simulink model "PNEUMA"  (R2023b)
settings: Solver=ode23tb  StartTime=0  StopTime=3600  FixedStep=0.001  MaxStep=time_step_new  RelTol=0.01  EnableMultiTasking=on
values from neighbouring files (symbols this model uses):
  A = 20.9    [Gas_Exchange_IC.m]    (also in getPneumonia.m = (LF1-LF2)/(1-exp(Rresolve*(t2(end)-t2(1)))))
  a1 = 0.3836    [Dissociation_Spencer_IC.m]    (also in Gas_Exchange_IC.m; Respiratory_IC.m)
  a2 = 1.819    [Dissociation_Spencer_IC.m]    (also in Gas_Exchange_IC.m; Respiratory_IC.m)
  alpha1 = 0.02598    [Dissociation_Spencer_IC.m]    (also in Gas_Exchange_IC.m; Respiratory_IC.m)
  alpha2 = 0.05591    [Dissociation_Spencer_IC.m]    (also in Gas_Exchange_IC.m; Respiratory_IC.m)
  B = 92.8    [Gas_Exchange_IC.m]    (also in getPneumonia.m = LungFunction(end)-A)
  beta1 = 0.012275    [Dissociation_Spencer_IC.m]    (also in Gas_Exchange_IC.m; Respiratory_IC.m)
  beta2 = 0.03255    [Dissociation_Spencer_IC.m]    (also in Gas_Exchange_IC.m; Respiratory_IC.m)
  C = 10570    [Gas_Exchange_IC.m]
  C1 = 9    [Dissociation_Spencer_IC.m]    (also in Gas_Exchange_IC.m; Respiratory_IC.m)
  C2 = 87.00    (= 87)    [Dissociation_Spencer_IC.m]    (also in Gas_Exchange_IC.m; Respiratory_IC.m)
  Circadian_Period = 24    [Respiratory_IC.m]    (also in State_UA_Khoo_IC.m)
  CvCO2IC = 0.5116    [Body_Khoo_IC.m]    (also in Gas_Exchange_IC.m; Respiratory_IC.m = 0.5247)
  CvO2IC = 0.1672    [Body_Khoo_IC.m]    (also in Gas_Exchange_IC.m; Respiratory_IC.m = 0.1639)
  D = -5.251    [Gas_Exchange_IC.m]
  Dead1CO2IC = 0.1020    (= 0.102)    [Dead_Space_Khoo_IC.m]    (also in Gas_Exchange_IC.m; Respiratory_IC.m = 39.5616)
  Dead1O2IC = 149.8824    [Dead_Space_Khoo_IC.m]    (also in Gas_Exchange_IC.m; Respiratory_IC.m = 104.3637)
  Dead2CO2IC = 0.5274    [Dead_Space_Khoo_IC.m]    (also in Gas_Exchange_IC.m; Respiratory_IC.m = 39.6736)
  Dead2O2IC = 149.3923    [Dead_Space_Khoo_IC.m]    (also in Gas_Exchange_IC.m; Respiratory_IC.m = 104.2258)
  Dead3CO2IC = 2.2996    [Dead_Space_Khoo_IC.m]    (also in Gas_Exchange_IC.m; Respiratory_IC.m = 39.8127)
  Dead3O2IC = 147.3503    [Dead_Space_Khoo_IC.m]    (also in Gas_Exchange_IC.m; Respiratory_IC.m = 104.0505)
  Dead4CO2IC = 8.2293    [Dead_Space_Khoo_IC.m]    (also in Gas_Exchange_IC.m; Respiratory_IC.m = 40.0061)
  Dead4O2IC = 140.5179    [Dead_Space_Khoo_IC.m]    (also in Gas_Exchange_IC.m; Respiratory_IC.m = 103.8005)
  Dead5CO2IC = 22.0757    [Dead_Space_Khoo_IC.m]    (also in Gas_Exchange_IC.m; Respiratory_IC.m = 40.3359)
  Dead5O2IC = 124.5641    [Dead_Space_Khoo_IC.m]    (also in Gas_Exchange_IC.m; Respiratory_IC.m = 103.3579)
  DtotalIC = 0.3    [NeuroMuscular_IC.m]    (also in Respiratory_IC.m = 0.32)
  E_CW = 5    [Pleural_Schuessler_IC.m]    (also in Pmus_Flow_Younes_IC.m; Resp_Mech_IC.m; Respiratory_IC.m)
  E_L = 5    [Pleural_Schuessler_IC.m]    (also in Pmus_Flow_Younes_IC.m; Resp_Mech_IC.m; Respiratory_IC.m)
  fc = 0.4/60    (= 0.00666666666667)    [Respiratory_IC.m]    (also in State_UA_Khoo_IC.m)
  fcs_max = 47.78    [Cardiovascular_IC.m]    (also in Reflex_Ursino_IC.m)
  fcs_min = 2.52    [Cardiovascular_IC.m]    (also in Reflex_Ursino_IC.m)
  fcs_zero = 25    [Respiratory_IC.m]
  FlowIC = 0    [Pmus_Flow_Younes_IC.m]    (also in Resp_Mech_IC.m; Respiratory_IC.m)
  fp_inf = 6.3    [Respiratory_IC.m]
  fp_zero = 3.2    [Respiratory_IC.m]
  fs_inf = 2.10    (= 2.1)    [Respiratory_IC.m]
  fs_zero = 16.11    [Respiratory_IC.m]
  ftbs_min = 0.1    [Cardiovascular_IC.m]    (also in SA_Node_Ursino_IC.m)
  gc = 0.008/60    (= 0.000133333333333)    [Respiratory_IC.m]    (also in State_UA_Khoo_IC.m)
  h = 0.0183    [Brain_Khoo_IC.m]    (also in Gas_Exchange_IC.m; Respiratory_IC.m)
  HP_basal = 0.58    [Cardiovascular_IC.m]    (also in SA_Node_Ursino_IC.m)
  Ic = 45    [Gas_Exchange_IC.m]    (also in Respiratory_IC.m; Vent_Drive_Khoo_IC.m)
  IpCO2 = 38    [Gas_Exchange_IC.m]    (also in Respiratory_IC.m; Vent_Drive_Khoo_IC.m)
  IpO2 = 102.4    [Gas_Exchange_IC.m]    (also in Respiratory_IC.m; Vent_Drive_Khoo_IC.m)
  K1 = 13    [Dissociation_Spencer_IC.m]    (also in Gas_Exchange_IC.m; Respiratory_IC.m)
  K2 = 194.4    [Dissociation_Spencer_IC.m]    (also in Gas_Exchange_IC.m; Respiratory_IC.m)
  k_cs = 11.758    [Cardiovascular_IC.m]    (also in Reflex_Ursino_IC.m)
  k_p = 7.06    [Respiratory_IC.m]
  k_s = 0.07    [Respiratory_IC.m]
  lambda = 863    [Gas_Exchange_IC.m]    (also in Lungs_Khoo_IC.m; Respiratory_IC.m)
  Mech_Vent_pressure = 17    [Mech_vent_test.m]
  MRbCO2 = 0.0517    [Brain_Khoo_IC.m]    (also in Gas_Exchange_IC.m; Respiratory_IC.m)
  MRCO2 = 0.0033    [Body_Khoo_IC.m]    (also in Gas_Exchange_IC.m; Respiratory_IC.m)
  MRO2 = 0.0038    [Body_Khoo_IC.m]    (also in Gas_Exchange_IC.m; Respiratory_IC.m)
  NM_block_gain = 1    [Mech_vent_test.m]
  PACO2_delayIC = 39.6041    [Cardio_Mix_Lange_IC.m]    (also in Gas_Exchange_IC.m; Respiratory_IC.m = 40.4448)
  PaCO2firstIC = 0.2150    (= 0.215)    [Cardio_Mix_Lange_IC.m]    (also in Gas_Exchange_IC.m; Respiratory_IC.m = -0.2465)
  PACO2IC = 37.1484    [Gas_Exchange_IC.m]    (also in Lungs_Khoo_IC.m; Respiratory_IC.m = 40.9432)
  PaCO2secondIC = 38.4577    [Cardio_Mix_Lange_IC.m]    (also in Gas_Exchange_IC.m; Respiratory_IC.m = 40.3928)
  PAO2_delayIC = 103.8436    [Cardio_Mix_Lange_IC.m]    (also in Gas_Exchange_IC.m; Respiratory_IC.m = 103.1223)
  PaO2firstIC = -0.2838    [Cardio_Mix_Lange_IC.m]    (also in Gas_Exchange_IC.m; Respiratory_IC.m = 0.3557)
  PAO2IC = 107.1983    [Gas_Exchange_IC.m]    (also in Lungs_Khoo_IC.m; Respiratory_IC.m = 102.5153)
  PaO2secondIC = 105.4828    [Cardio_Mix_Lange_IC.m]    (also in Gas_Exchange_IC.m; Respiratory_IC.m = 103.1435)
  PbCO2IC = 48.2858    [Brain_Khoo_IC.m]    (also in Gas_Exchange_IC.m; Respiratory_IC.m = 48.5383)
  PICO2 = 0    [Dead_Space_Khoo_IC.m]    (also in Gas_Exchange_IC.m; Respiratory_IC.m)
  PIO2 = 150    [Dead_Space_Khoo_IC.m]    (also in Gas_Exchange_IC.m; Respiratory_IC.m)
  PIO2_change = -90    [Mech_vent_test.m]    (also in Respiratory_IC.m = 0)
  Pn = 90    [Cardiovascular_IC.m]    (also in Reflex_Ursino_IC.m)
  Pt_frcIC1 = 0    [Pmus_Flow_Younes_IC.m]    (also in Resp_Mech_IC.m; Respiratory_IC.m)
  Pt_frcIC2 = 0    [Pmus_Flow_Younes_IC.m]    (also in Resp_Mech_IC.m; Respiratory_IC.m)
  QdBo = 0.8333    [Brain_Khoo_IC.m]    (also in Gas_Exchange_IC.m; Respiratory_IC.m)
  R_AW = 1.27    [Pleural_Schuessler_IC.m]    (also in Pmus_Flow_Younes_IC.m; Resp_Mech_IC.m; Respiratory_IC.m)
  R_CW = 1.03    [Pleural_Schuessler_IC.m]    (also in Pmus_Flow_Younes_IC.m; Resp_Mech_IC.m; Respiratory_IC.m)
  R_L = 1.69    [Pleural_Schuessler_IC.m]    (also in Pmus_Flow_Younes_IC.m; Resp_Mech_IC.m; Respiratory_IC.m)
  RC = 0.06    [Pleural_Schuessler_IC.m]    (also in Pmus_Flow_Younes_IC.m; Resp_Mech_IC.m; Respiratory_IC.m)
  rc = 0.2/60    (= 0.00333333333333)    [Respiratory_IC.m]    (also in State_UA_Khoo_IC.m)
  SbCO2 = 0.3600    (= 0.36)    [Brain_Khoo_IC.m]    (also in Gas_Exchange_IC.m; Respiratory_IC.m)
  SCO2 = 0.0043    [Brain_Khoo_IC.m]    (also in Gas_Exchange_IC.m; Respiratory_IC.m)
  SWAo = 0.007    [Respiratory_IC.m]    (also in State_UA_Khoo_IC.m)
  T1 = 1    [Cardio_Mix_Lange_IC.m]    (also in Gas_Exchange_IC.m; Respiratory_IC.m)
  T2 = 2    [Cardio_Mix_Lange_IC.m]    (also in Gas_Exchange_IC.m; Respiratory_IC.m)
  t_end_new = 4*24*60*60    (= 345600)    [Mech_vent_test.m]
  t_end_UA = 0    [Respiratory_IC.m]    (also in State_UA_Khoo_IC.m)
  t_Mech_Vent_duration = 0    [Mech_vent_test.m]
  t_Mech_Vent_start = 0    [Mech_vent_test.m]
  t_Mueller_duration = 0    [NeuroMuscular_IC.m]
  t_Mueller_insp = 0    [NeuroMuscular_IC.m]
  t_Mueller_start = 0    [NeuroMuscular_IC.m]
  t_NM_block_duration = 0    [Mech_vent_test.m]
  t_NM_block_start = 0    [Mech_vent_test.m]
  t_O2_duration = 0    [Mech_vent_test.m]    (also in Respiratory_IC.m)
  t_O2_start = 0    [Mech_vent_test.m]    (also in Respiratory_IC.m)
  t_start_new = 0    [Mech_vent_test.m]
  t_start_UA = 0    [Respiratory_IC.m]    (also in State_UA_Khoo_IC.m)
  t_valsalva_duration = 0    [NeuroMuscular_IC.m]
  t_valsalva_insp = 0    [NeuroMuscular_IC.m]
  t_valsalva_start = 0    [NeuroMuscular_IC.m]
  time_step = time_step    [acquire_data.m]    (also in acquire_data_save.m)
  VC = 5    [Pmus_Flow_Younes_IC.m]    (also in Resp_Mech_IC.m; Respiratory_IC.m)
  Vdead1 = 0.03    [Dead_Space_Khoo_IC.m]    (also in Gas_Exchange_IC.m; Respiratory_IC.m)
  Vdead2 = 0.03    [Dead_Space_Khoo_IC.m]    (also in Gas_Exchange_IC.m; Respiratory_IC.m)
  Vdead3 = 0.03    [Dead_Space_Khoo_IC.m]    (also in Gas_Exchange_IC.m; Respiratory_IC.m)
  Vdead4 = 0.03    [Dead_Space_Khoo_IC.m]    (also in Gas_Exchange_IC.m; Respiratory_IC.m)
  Vdead5 = 0.03    [Dead_Space_Khoo_IC.m]    (also in Gas_Exchange_IC.m; Respiratory_IC.m)
  Ventilator_rate = 12    [Mech_vent_test.m]
  VTCO2 = 15    [Body_Khoo_IC.m]    (also in Gas_Exchange_IC.m; Respiratory_IC.m)
  VtIC = 0    [Pmus_Flow_Younes_IC.m]    (also in Resp_Mech_IC.m; Respiratory_IC.m)
  VTO2 = 6    [Body_Khoo_IC.m]    (also in Gas_Exchange_IC.m; Respiratory_IC.m)
  Z = 0.0227    [Dissociation_Spencer_IC.m]    (also in Gas_Exchange_IC.m; Respiratory_IC.m)
undefined symbols (not defined in the file or in its folder): A_0_ua, alpha_E_FFA_Heart, alpha_E_FFA_muscle, alpha_E_GLC_Heart, alpha_E_GLC_muscle, alpha_E_GLY_muscle, alpha_E_PYR_muscle, alpha_E_TGL_adipose, alpha_E_TGL_GI, alpha_E_TGL_Heart, alpha_E_TGL_muscle, Arousal_UAIC, C_ua_awake, Cbp, Cbv, Ce_0, Cep, Cev, Chp, Chv, Cla, Clamp_class, Cmp, Cmv, Cpa, CPAP_pressure, Cpp, Cpv, Cra, Csa, Csp, Csv, CvbO2_n, CvhO2_n, CvmO2_n, DAY, delay, DietBlock, Dx, Fb, fchemo_max, fchemo_min, fchemoIC, flsIC, Ftas_I0, ftas_min, ftas_r0, FVC_activation, gain_E, Gamma, Gas_sleep, Gas_sleepM, Gb, Gblock, GbO2, Gbs_sleep, gcc_sa, gcc_sb, gcc_sp, Gclamp ... (+144)
libraries: simulink x4, dspstat3 x4, simulink_extras x2
(part 7 of 8)

== system PNEUMA/Metabolic Control/Epinephrine Regulation on Heart and Muscle/Epi Modulation/Muscle ==
  Ce(t) : Inport
  Add : Sum  Inputs=+++++
  Fcn{,1..4} (5 alike) : Fcn  Expr=u(2) * ( 1+ u(4) * (u(1) - u(3))^2/( u(5)+(u(1) - u(3))^2 ))
  Muscle: FFA_to_ACoA : Constant  Value=[V_0_FFA_muscle, Ce_0, lamda_E_FFA_muscle, alpha_E_FFA_muscle]
  Muscle: GLC_to_G6P : Constant  Value=[V_0_GLC_muscle, Ce_0, lamda_E_GLC_muscle, alpha_E_GLC_muscle]
  Muscle: GLY_to_G6P : Constant  Value=[V_0_GLY_muscle, Ce_0, lamda_E_GLY_muscle, alpha_E_GLY_muscle]
  Muscle: PYR_to_ALA : Constant  Value=[V_0_PYR_muscle, Ce_0, lamda_E_PYR_muscle, alpha_E_PYR_muscle]
  Muscle: TGL_to_FFA : Constant  Value=[V_0_TGL_muscle, Ce_0, lamda_E_TGL_muscle, alpha_E_TGL_muscle]
  Mux{,1..2,4..5} (5 alike) : Mux  Inputs=2
  Mux3 : Mux  Inputs=5
  Epi on Muscle (Fluxes) : Outport
  Epi on Muscle(Sum) : Outport  Port=2
  wires:
  Ce(t)/1 -> Mux/1, Mux1/1, Mux2/1, Mux4/1, Mux5/1
  Muscle: GLC_to_G6P/1 -> Mux/2
  Mux/1 -> Fcn/1
  Muscle: GLY_to_G6P/1 -> Mux1/2
  Mux1/1 -> Fcn1/1
  Muscle: FFA_to_ACoA/1 -> Mux2/2
  Mux2/1 -> Fcn2/1
  Fcn/1 -> Mux3/1, Add/1
  Fcn1/1 -> Mux3/2, Add/2
  Muscle: TGL_to_FFA/1 -> Mux4/2
  Mux4/1 -> Fcn3/1
  Fcn3/1 -> Mux3/5, Add/5
  Fcn2/1 -> Mux3/3, Add/3
  Mux3/1 -> Epi on Muscle (Fluxes)/1
  Add/1 -> Epi on Muscle(Sum)/1
  Muscle: PYR_to_ALA/1 -> Mux5/2
  Mux5/1 -> Fcn4/1
  Fcn4/1 -> Mux3/4, Add/4

== system PNEUMA/Metabolic Control/Glucose-Insulin-FFA Minimal Model/Saving deltaFtas_WalphaSYMP/Switch Case Action Subsystem ==
  In1 : Inport
  Action Port : ActionPort  ActionPortLabel=case [ 0 ]:
  To File : ToFile  Filename=deltaFtas1.mat  MatrixName=deltaFtas  SampleTime=sampletime
  wires:
  In1/1 -> To File/1

== system PNEUMA/Metabolic Control/Glucose-Insulin-FFA Minimal Model/Saving deltaFtas_WalphaSYMP/Switch Case Action Subsystem1 ==
  In1 : Inport
  Action Port : ActionPort  ActionPortLabel=case [ 1 ]:
  To File : ToFile  Filename=deltaFtas2.mat  MatrixName=deltaFtas  SampleTime=sampletime
  wires:
  In1/1 -> To File/1

== system PNEUMA/Metabolic Control/Glucose-Insulin-FFA Minimal Model/Saving deltaFtas_WalphaSYMP/Switch Case Action Subsystem2 ==
  In1 : Inport
  Action Port : ActionPort  ActionPortLabel=case [ 2 ]:
  To File : ToFile  Filename=deltaFtas3.mat  MatrixName=deltaFtas  SampleTime=sampletime
  wires:
  In1/1 -> To File/1

== system PNEUMA/Metabolic Control/Glucose-Insulin-FFA Minimal Model/Saving deltaFtas_WalphaSYMP/Switch Case Action Subsystem3 ==
  In1 : Inport
  Action Port : ActionPort  ActionPortLabel=default:
  To File : ToFile  Filename=deltaFtas10.mat  MatrixName=deltaFtas  SampleTime=sampletime
  wires:
  In1/1 -> To File/1

== system PNEUMA/Metabolic Control/Glucose-Insulin-FFA Minimal Model/Saving deltaFtas_WalphaSYMP/Switch Case Action Subsystem4 ==
  In1 : Inport
  Action Port : ActionPort  ActionPortLabel=case [ 3 ]:
  To File : ToFile  Filename=deltaFtas4.mat  MatrixName=deltaFtas  SampleTime=sampletime
  wires:
  In1/1 -> To File/1

== system PNEUMA/Metabolic Control/Glucose-Insulin-FFA Minimal Model/Saving deltaFtas_WalphaSYMP/Switch Case Action Subsystem5 ==
  In1 : Inport
  Action Port : ActionPort  ActionPortLabel=case [ 4 ]:
  To File : ToFile  Filename=deltaFtas5.mat  MatrixName=deltaFtas  SampleTime=sampletime
  wires:
  In1/1 -> To File/1

== system PNEUMA/Metabolic Control/Glucose-Insulin-FFA Minimal Model/Saving deltaFtas_WalphaSYMP/Switch Case Action Subsystem6 ==
  In1 : Inport
  Action Port : ActionPort  ActionPortLabel=case [ 5 ]:
  To File : ToFile  Filename=deltaFtas6.mat  MatrixName=deltaFtas  SampleTime=sampletime
  wires:
  In1/1 -> To File/1

== system PNEUMA/Metabolic Control/Glucose-Insulin-FFA Minimal Model/Saving deltaFtas_WalphaSYMP/Switch Case Action Subsystem7 ==
  In1 : Inport
  Action Port : ActionPort  ActionPortLabel=case [ 6 ]:
  To File : ToFile  Filename=deltaFtas7.mat  MatrixName=deltaFtas  SampleTime=sampletime
  wires:
  In1/1 -> To File/1

== system PNEUMA/Metabolic Control/Glucose-Insulin-FFA Minimal Model/Saving deltaFtas_WalphaSYMP/Switch Case Action Subsystem8 ==
  In1 : Inport
  Action Port : ActionPort  ActionPortLabel=case [ 7 ]:
  To File : ToFile  Filename=deltaFtas8.mat  MatrixName=deltaFtas  SampleTime=sampletime
  wires:
  In1/1 -> To File/1

== system PNEUMA/Metabolic Control/Glucose-Insulin-FFA Minimal Model/Saving deltaFtas_WalphaSYMP/Switch Case Action Subsystem9 ==
  In1 : Inport
  Action Port : ActionPort  ActionPortLabel=case [ 8 ]:
  To File : ToFile  Filename=deltaFtas9.mat  MatrixName=deltaFtas  SampleTime=sampletime
  wires:
  In1/1 -> To File/1

== system PNEUMA/Respiratory System/Gas Exchange/BODY TISSUES COMPARTMENT/Body Tissues Compartment for CO2 ==
  CaCO2 : Inport
  Qt : Inport  Port=2
  SI Sleep Wake State Index : Inport  Port=3
  Fcn : Fcn  Expr=MRCO2*(0.375*(1-0.4*u)+0.625)
  Fcn -5 blocks : Fcn  Expr=( u(1) + ( u(2) * u(3)) ) /VTCO2
  Integrator : Integrator  InitialCondition=CvCO2IC
  Mux : Mux  Inputs=3
  Sum1 : Sum  Inputs=+-  InputSameDT=on  SaturateOnIntegerOverflow=on  OutDataTypeStr=Inherit: Same as first input
  CvCO2 : Outport
  tag scope: CvCO2IC=global
  wires:
  SI Sleep Wake State Index/1 -> Fcn/1
  CaCO2/1 -> Sum1/1
  Fcn -5 blocks/1 -> Integrator/1
  Integrator/1 -> [CvCO2IC], Sum1/2, CvCO2/1
  Mux/1 -> Fcn -5 blocks/1
  Fcn/1 -> Mux/1
  Qt/1 -> Mux/2
  Sum1/1 -> Mux/3

== system PNEUMA/Respiratory System/Gas Exchange/BODY TISSUES COMPARTMENT/Body Tissues Compartment for O2 ==
  Qt : Inport
  SI Sleep Wake State Index : Inport  Port=2
  CaO2 : Inport  Port=3
  Fcn : Fcn  Expr=MRO2*(0.375*(1-0.4*u)+0.625)
  Fcn -5 blocks : Fcn  Expr=( -u(1) + ( u(2) * u(3)) ) /VTO2
  Integrator : Integrator  InitialCondition=CvO2IC
  Mux : Mux  Inputs=3
  Sum1 : Sum  Inputs=+-  InputSameDT=on  SaturateOnIntegerOverflow=on  OutDataTypeStr=Inherit: Same as first input
  CVO2 : Outport
  tag scope: CvO2IC=global
  wires:
  SI Sleep Wake State Index/1 -> Fcn/1
  Qt/1 -> Mux/2
  Sum1/1 -> Mux/3
  CaO2/1 -> Sum1/1
  Fcn -5 blocks/1 -> Integrator/1
  Integrator/1 -> [CvO2IC], Sum1/2, CVO2/1
  Mux/1 -> Fcn -5 blocks/1
  Fcn/1 -> Mux/1

== system PNEUMA/Respiratory System/Gas Exchange/Cardiovascular Mixing and Convection/CO2 Cardiovascular Mixing and Convection Effects ==
  PACO2 : Inport
  Q : Inport  Port=2
  Lung-Chemoreceptor Delay Volume : Inport  Port=3
  1/(T1*T2) : Gain  Gain=1/(T1*T2)  SaturateOnIntegerOverflow=on  OutDataTypeStr=Inherit: Same as input  ParamDataTypeStr=Inherit: Same as input
  Integrator : Integrator  InitialCondition=PaCO2firstIC
  Integrator1 : Integrator  InitialCondition=PaCO2secondIC
  PACO2 delay : VariableTransportDelay  MaximumDelay=100  InitialOutput=PACO2_delayIC  MaximumPoints=22528
  Product1 : Product  Inputs=*/  InputSameDT=on  SaturateOnIntegerOverflow=on  OutDataTypeStr=Inherit: Same as first input
  Sum : Sum  Inputs=--+  InputSameDT=on  SaturateOnIntegerOverflow=on  OutDataTypeStr=Inherit: Same as first input
  T1+T2 : Gain  Gain=T1+T2  SaturateOnIntegerOverflow=on  OutDataTypeStr=Inherit: Same as input  ParamDataTypeStr=Inherit: Same as input
  PaCO2 : Outport
  tag scope: PACO2_delayIC=global, PaCO2firstIC=global, PaCO2secondIC=global
  wires:
  T1+T2/1 -> Sum/1
  Integrator/1 -> T1+T2/1, Integrator1/1, [PaCO2firstIC]
  Sum/1 -> 1/(T1*T2)/1
  1/(T1*T2)/1 -> Integrator/1
  Integrator1/1 -> Sum/2, [PaCO2secondIC], PaCO2/1
  PACO2/1 -> PACO2 delay/1
  PACO2 delay/1 -> [PACO2_delayIC], Sum/3
  Product1/1 -> PACO2 delay/2
  Lung-Chemoreceptor Delay Volume/1 -> Product1/1
  Q/1 -> Product1/2

== system PNEUMA/Respiratory System/Gas Exchange/Cardiovascular Mixing and Convection/O2 Cardiovascular Mixing and Convection Effects ==
  note: Warning: Division by zero in block 'pneuma_cardiovascular/Respiratory_System/Gas Exchange/Cardiovascular Mixing and Convection/O2 Cardiovascular Mixing and Convection Effects/PAO2 Save Subsystem/Product1'.
  Q : Inport
  PAO2 : Inport  Port=2
  Lung-Chemoreceptor Delay Volume : Inport  Port=3
  1/(T1*T2) : Gain  Gain=1/(T1*T2)  SaturateOnIntegerOverflow=on  OutDataTypeStr=Inherit: Same as input  ParamDataTypeStr=Inherit: Same as input
  Integrator : Integrator  InitialCondition=PaO2firstIC
  Integrator1 : Integrator  InitialCondition=PaO2secondIC
  PAO2 delay : VariableTransportDelay  MaximumDelay=100  InitialOutput=PAO2_delayIC  MaximumPoints=22528
  Product1 : Product  Inputs=*/  InputSameDT=on  SaturateOnIntegerOverflow=on  OutDataTypeStr=Inherit: Same as first input
  Sum : Sum  Inputs=+--  InputSameDT=on  SaturateOnIntegerOverflow=on  OutDataTypeStr=Inherit: Same as first input
  T1+T2 : Gain  Gain=T1+T2  SaturateOnIntegerOverflow=on  OutDataTypeStr=Inherit: Same as input  ParamDataTypeStr=Inherit: Same as input
  PaO2 : Outport
  tag scope: PAO2_delayIC=global, PaO2firstIC=global, PaO2secondIC=global
  wires:
  1/(T1*T2)/1 -> Integrator/1
  Sum/1 -> 1/(T1*T2)/1
  Integrator/1 -> Integrator1/1, T1+T2/1, [PaO2firstIC]
  Integrator1/1 -> Sum/2, PaO2/1, [PaO2secondIC]
  T1+T2/1 -> Sum/3
  Product1/1 -> PAO2 delay/2
  PAO2/1 -> PAO2 delay/1
  PAO2 delay/1 -> [PAO2_delayIC], Sum/1
  Lung-Chemoreceptor Delay Volume/1 -> Product1/1
  Q/1 -> Product1/2

== system PNEUMA/Respiratory System/Gas Exchange/DEAD SPACE/CO2 DEAD SPACE ==
  PACO2 : Inport
  Flow : Inport  Port=2
  Constant : Constant  Value=PICO2
  Pd(1)CO2 : Subsystem
  Pd(2)CO2 : Subsystem
  Pd(3)CO2 : Subsystem
  Pd(4)CO2 : Subsystem
  Pd(5)CO2 : Subsystem
  Pd5CO2 : Outport
  tag scope: BreathCO2=global
  wires:
  Pd(4)CO2/1(Pd(4)CO2) -> Pd(3)CO2/3(Pd(4)CO2), Pd(5)CO2/1(Pd(4)CO2)
  Pd(3)CO2/1(Pd(3)CO2) -> Pd(4)CO2/1(Pd(3)CO2), Pd(2)CO2/3(Pd(3)CO2)
  Pd(2)CO2/1(Pd(2)CO2) -> Pd(3)CO2/1(Pd(2)CO2), Pd(1)CO2/3(Pd(2)CO2)
  Pd(1)CO2/1(Pd(1)CO2) -> [BreathCO2], Pd(2)CO2/1(Pd(1)CO2)
  Flow/1 -> Pd(1)CO2/2(Flow), Pd(2)CO2/2(Flow), Pd(4)CO2/2(Flow), Pd(5)CO2/2(Flow), Pd(3)CO2/2(Flow)
  PACO2/1 -> Pd(5)CO2/3(PACO2)
  Pd(5)CO2/1(Pd(5)CO2) -> Pd5CO2/1, Pd(4)CO2/3(Pd(5)CO2)
  Constant/1 -> Pd(1)CO2/1(PICO2)

== system PNEUMA/Respiratory System/Gas Exchange/DEAD SPACE/O2 DEAD SPACE ==
  Flow : Inport
  PAO2 : Inport  Port=2
  Pd(1)O2 : Subsystem
  Pd(2)O2 : Subsystem
  Pd(3)O2 : Subsystem
  Pd(4)O2 : Subsystem
  Pd(5)O2 : Subsystem
  Pd5O2 : Outport
  wires:
  Pd(4)O2/1(Pd(4)O2) -> Pd(3)O2/3(Pd(4)O2), Pd(5)O2/1(Pd(4)O2)
  Pd(3)O2/1(Pd(3)O2) -> Pd(4)O2/1(Pd(3)O2), Pd(2)O2/3(Pd(3)O2)
  Pd(2)O2/1(Pd(2)O2) -> Pd(3)O2/1(Pd(2)O2), Pd(1)O2/3(Pd(2)O2)
  Pd(1)O2/1(Pd(1)O2) -> Pd(2)O2/1(Pd(1)O2)
  PAO2/1 -> Pd(5)O2/3(PAO2)
  Flow/1 -> Pd(4)O2/2(Flow), Pd(5)O2/2(Flow), Pd(2)O2/2(Flow), Pd(1)O2/2(Flow), Pd(3)O2/2(Flow)
  Pd(5)O2/1(Pd(5)O2) -> Pd5O2/1, Pd(4)O2/3(Pd(5)O2)
  [PIO2] -> Pd(1)O2/1(PIO2)

== system PNEUMA/Respiratory System/Gas Exchange/GAS EXCHANGE IN THE LUNGS/CO2 Gas Exchange in the Lungs ==
  CaCO2 : Inport
  CVCO2 : Inport  Port=2
  Pd5CO2 : Inport  Port=3
  Vt - Tidal Volume : Inport  Port=4
  Flow : Inport  Port=5
  "Q " : Inport  Port=6
  Constant : Constant  Value=lambda
  Fcn -11 blocks : Fcn  Expr=(((u(2) >=0) * u(2) * u(1) + (u(2) <0) * 0 ) + (u(3) - u(4)) *u(5) * ( u(7)*(1-s) ) )/( u(6)+VLCO2)
  From Workspace : FromWorkspace  VariableName=LungFunction
  Integrator : Integrator  InitialCondition=PACO2IC
  Mux : Mux  Inputs=7
  Product : Product  Inputs=*/
  sum1 : Sum  Inputs=-+  InputSameDT=on  SaturateOnIntegerOverflow=on  OutDataTypeStr=Inherit: Same as first input
  PACO2 : Outport
  tag scope: PACO2IC=global
  wires:
  "Q "/1 -> Mux/5
  CVCO2/1 -> Mux/3
  CaCO2/1 -> Mux/4
  Fcn -11 blocks/1 -> Integrator/1
  Integrator/1 -> [PACO2IC], PACO2/1, sum1/1
  Pd5CO2/1 -> sum1/2
  Mux/1 -> Fcn -11 blocks/1
  sum1/1 -> Mux/1
  Flow/1 -> Mux/2
  Vt - Tidal Volume/1 -> Mux/6
  Product/1 -> Mux/7
  Constant/1 -> Product/1
  From Workspace/1 -> Product/2

== system PNEUMA/Respiratory System/Gas Exchange/GAS EXCHANGE IN THE LUNGS/O2 Gas Exchange in the Lungs ==
  Vt - Tidal Volume : Inport
  Flow : Inport  Port=2
  Q : Inport  Port=3
  CaO2 : Inport  Port=4
  CVO2 : Inport  Port=5
  Pd5O2 : Inport  Port=6
  Constant : Constant  Value=lambda
  Fcn -11 blocks : Fcn  Expr=(((u(2) >=0) * u(2) * u(1) + (u(2) <0) * 0 ) + (u(4) - u(5)) *u(3) * ( u(7)*(1-s) ) )/( u(6)+VLO2 )
  From Workspace : FromWorkspace  VariableName=LungFunction
  Integrator : Integrator  InitialCondition=PAO2IC  LimitOutput=on  LowerSaturationLimit=0
  Mux : Mux  Inputs=7
  Product : Product  Inputs=*/
  Sum2 : Sum  Inputs=-+  InputSameDT=on  SaturateOnIntegerOverflow=on  OutDataTypeStr=Inherit: Same as first input
  PAO2 : Outport
  tag scope: LungFunction=global, PAO2IC=global
  wires:
  Integrator/1 -> PAO2/1, [PAO2IC], Sum2/1
  Fcn -11 blocks/1 -> Integrator/1
  Pd5O2/1 -> Sum2/2
  Mux/1 -> Fcn -11 blocks/1
  Sum2/1 -> Mux/1
  Flow/1 -> Mux/2
  Q/1 -> Mux/3
  CVO2/1 -> Mux/4
  CaO2/1 -> Mux/5
  Vt - Tidal Volume/1 -> Mux/6
  Product/1 -> Mux/7
  Constant/1 -> Product/1
  From Workspace/1 -> [LungFunction], Product/2

== system PNEUMA/Respiratory System/Respiratory_Mechanics/Pleural_Pressure1/Pa ==
  "Flow " : Inport
  "Pao " : Inport  Port=2
  Fcn : Fcn  Expr=(u>=0)*u * (kaw1 + abs( (u>=0)*u) *kaw2)
  Fcn1 : Fcn  Expr=(u>=0)*u
  Sum2 : Sum  Inputs=+-  InputSameDT=on  SaturateOnIntegerOverflow=on  OutDataTypeStr=Inherit: Same as first input
  "Pa " : Outport
  wires:
  "Flow "/1 -> Fcn/1
  "Pao "/1 -> Sum2/1
  Sum2/1 -> Fcn1/1
  Fcn/1 -> Sum2/2
  Fcn1/1 -> "Pa "/1

== system PNEUMA/Respiratory System/Respiratory_Mechanics/Pleural_Pressure1/Pcw ==
  Vt : Inport
  Flow : Inport  Port=2
  Fcn : Fcn  Expr=(u>=0)*u
  Pcw_0 : Constant  Value=-1
  Product3 : Product  InputSameDT=on  SaturateOnIntegerOverflow=on  OutDataTypeStr=Inherit: Same as first input
  Product4 : Product  InputSameDT=on  SaturateOnIntegerOverflow=on  OutDataTypeStr=Inherit: Same as first input
  Sum3 : Sum  Inputs=+++  InputSameDT=on  SaturateOnIntegerOverflow=on  OutDataTypeStr=Inherit: Same as first input
  elastance : Constant  Value=E_CW
  "resistance " : Constant  Value=R_CW
  "Pcw " : Outport
  wires:
  Fcn/1 -> Product3/2
  Vt/1 -> Product4/1
  elastance/1 -> Product4/2
  Sum3/1 -> "Pcw "/1
  Product4/1 -> Sum3/2
  Flow/1 -> Fcn/1
  Product3/1 -> Sum3/1
  "resistance "/1 -> Product3/1
  Pcw_0/1 -> Sum3/3

== system PNEUMA/Respiratory System/Respiratory_Mechanics/Respiratory Muscles Activity1/Resp Muscle Reaction ==
  RespMus Drive : Inport
  Step Size : Inport  Port=2
  0.735539 : Gain
  Fcn : Fcn  Expr=u(1) + u(2) + (u(2) *u(5)/u(4) - u(3)+u(1)) * (exp(-u(4)/u(5)) - 1)
  Memory : Memory  InitialCondition=Pt_frcIC1  InheritSampleTime=on
  Memory1 : Memory  InitialCondition=Pt_frcIC2  InheritSampleTime=on  LinearizeMemory=on
  Mux : Mux  Inputs=5
  RC1 : Constant  Value=RC
  Sum4 : Sum  Inputs=+-  InputSameDT=on  SaturateOnIntegerOverflow=on  OutDataTypeStr=Inherit: Same as first input
  Pt_frc : Outport
  wires:
  RespMus Drive/1 -> Sum4/1, Memory/1
  Sum4/1 -> Mux/2
  RC1/1 -> Mux/5
  Step Size/1 -> Mux/4
  Memory1/1 -> Mux/1
  Memory/1 -> Sum4/2, Mux/3
  Mux/1 -> Fcn/1
  Fcn/1 -> 0.735539/1
  0.735539/1 -> Pt_frc/1, Memory1/1

== system PNEUMA/Respiratory System/Respiratory_Mechanics/Respiratory Muscles Activity1/flow generation ==
  "Cond " : Inport
  "Pao " : Inport  Port=2
  PE : Inport  Port=3
  "Po_vt " : Inport  Port=4
  b_vt : Inport  Port=5
  Vt : Inport  Port=6
  0.25 : Gain  Gain=0.25  SaturateOnIntegerOverflow=on  OutDataTypeStr=Inherit: Same as input  ParamDataTypeStr=Inherit: Same as input
  4 : Gain  Gain=4  SaturateOnIntegerOverflow=on  OutDataTypeStr=Inherit: Same as input  ParamDataTypeStr=Inherit: Same as input
  Gain3 : Gain  Gain=1/2  SaturateOnIntegerOverflow=on  OutDataTypeStr=Inherit: Same as input  ParamDataTypeStr=Inherit: Same as input
  Math Function : Math  Operator=square  SignedPower=on
  Math Function1 : Math  Operator=sqrt  SignedPower=on
  Memory3 : Memory  InitialCondition=FlowIC  InheritSampleTime=on
  Product : Product  InputSameDT=on  SaturateOnIntegerOverflow=on  OutDataTypeStr=Inherit: Same as first input
  Product1 : Product  InputSameDT=on  SaturateOnIntegerOverflow=on  OutDataTypeStr=Inherit: Same as first input
  Product2 : Product  Inputs=3  InputSameDT=on  SaturateOnIntegerOverflow=on  OutDataTypeStr=Inherit: Same as first input
  Sum4 : Sum  Inputs=+++-  InputSameDT=on  SaturateOnIntegerOverflow=on  OutDataTypeStr=Inherit: Same as first input
  Sum5 : Sum  InputSameDT=on  SaturateOnIntegerOverflow=on  OutDataTypeStr=Inherit: Same as first input
  Sum6 : Sum  Inputs=+-  InputSameDT=on  SaturateOnIntegerOverflow=on  OutDataTypeStr=Inherit: Same as first input
  Sum7 : Sum  Inputs=++--  InputSameDT=on  SaturateOnIntegerOverflow=on  OutDataTypeStr=Inherit: Same as first input
  Sum8 : Sum  Inputs=-+  InputSameDT=on  SaturateOnIntegerOverflow=on  OutDataTypeStr=Inherit: Same as first input
  elastance : Gain  Gain=(E_CW+E_L)  SaturateOnIntegerOverflow=on  OutDataTypeStr=Inherit: Same as input  ParamDataTypeStr=Inherit: Same as input
  total_resp conductance : Constant  Value=1/(R_AW+R_L+R_CW)*1.8
  Flow : Outport
  wires:
  0.25/1 -> Sum4/1
  total_resp conductance/1 -> Product1/2
  "Cond "/1 -> Product1/1
  Product1/1 -> 4/1, Product/1
  Gain3/1 -> Memory3/1
  Sum8/1 -> Gain3/1
  Sum5/1 -> Sum8/1, Math Function/1
  Math Function1/1 -> Sum8/2
  Sum6/1 -> Math Function1/1
  Product2/1 -> Sum6/2
  "Po_vt "/1 -> Sum7/4, 0.25/1
  "Pao "/1 -> Sum7/3, Sum4/4
  PE/1 -> Sum7/2, Sum4/3
  elastance/1 -> Sum7/1, Sum4/2
  Sum7/1 -> Product2/3
  b_vt/1 -> Product2/2, Sum5/2
  4/1 -> Product2/1
  Math Function/1 -> Sum6/1
  Product/1 -> Sum5/1
  Sum4/1 -> Product/2
  Vt/1 -> elastance/1
  Memory3/1 -> Flow/1

== system PNEUMA/Respiratory System/Respiratory_Mechanics/Respiratory Muscles Activity1/flow generation 1 ==
  Po_vt_1 : Inport
  Vt_1 : Inport  Port=2
  b_vt_1 : Inport  Port=3
  PE_1 : Inport  Port=4
  Pao_1 : Inport  Port=5
  "Cond " : Inport  Port=6
  0.25 : Gain  Gain=0.25  SaturateOnIntegerOverflow=on  OutDataTypeStr=Inherit: Same as input  ParamDataTypeStr=Inherit: Same as input
  4 : Gain  Gain=4  SaturateOnIntegerOverflow=on  OutDataTypeStr=Inherit: Same as input  ParamDataTypeStr=Inherit: Same as input
  Gain3 : Gain  Gain=0.5  SaturateOnIntegerOverflow=on  OutDataTypeStr=Inherit: Same as input  ParamDataTypeStr=Inherit: Same as input
  Math Function : Math  Operator=square  SignedPower=on
  Math Function1 : Math  Operator=sqrt  SignedPower=on
  Memory1 : Memory  InitialCondition=FlowIC  InheritSampleTime=on
  Product : Product  InputSameDT=on  SaturateOnIntegerOverflow=on  OutDataTypeStr=Inherit: Same as first input
  Product1 : Product  InputSameDT=on  SaturateOnIntegerOverflow=on  OutDataTypeStr=Inherit: Same as first input
  Product2 : Product  Inputs=3  InputSameDT=on  SaturateOnIntegerOverflow=on  OutDataTypeStr=Inherit: Same as first input
  Sum4 : Sum  Inputs=+++-  InputSameDT=on  SaturateOnIntegerOverflow=on  OutDataTypeStr=Inherit: Same as first input
  Sum5 : Sum  InputSameDT=on  SaturateOnIntegerOverflow=on  OutDataTypeStr=Inherit: Same as first input
  Sum6 : Sum  Inputs=+-  InputSameDT=on  SaturateOnIntegerOverflow=on  OutDataTypeStr=Inherit: Same as first input
  Sum7 : Sum  Inputs=++--  InputSameDT=on  SaturateOnIntegerOverflow=on  OutDataTypeStr=Inherit: Same as first input
  Sum8 : Sum  Inputs=-+  InputSameDT=on  SaturateOnIntegerOverflow=on  OutDataTypeStr=Inherit: Same as first input
  elastance : Gain  Gain=(E_CW+E_L)  SaturateOnIntegerOverflow=on  OutDataTypeStr=Inherit: Same as input  ParamDataTypeStr=Inherit: Same as input
  total_resp conductance : Constant  Value=1/(R_AW+R_L+R_CW)*1.8
  Flow_1 : Outport
  wires:
  Vt_1/1 -> elastance/1
  Sum4/1 -> Product/2
  Product/1 -> Sum5/1
  Math Function/1 -> Sum6/1
  4/1 -> Product2/1
  b_vt_1/1 -> Sum5/2, Product2/2
  Sum7/1 -> Product2/3
  elastance/1 -> Sum4/2, Sum7/1
  PE_1/1 -> Sum4/3, Sum7/2
  Pao_1/1 -> Sum4/4, Sum7/3
  Po_vt_1/1 -> 0.25/1, Sum7/4
  Product2/1 -> Sum6/2
  Sum6/1 -> Math Function1/1
  Math Function1/1 -> Sum8/2
  Sum5/1 -> Math Function/1, Sum8/1
  Sum8/1 -> Gain3/1
  Gain3/1 -> Memory1/1
  Product1/1 -> Product/1, 4/1
  "Cond "/1 -> Product1/1
  total_resp conductance/1 -> Product1/2
  0.25/1 -> Sum4/1
  Memory1/1 -> Flow_1/1

== system PNEUMA/Respiratory System/Sleep Mechanism/Saving CircadianProcess/Switch Case Action Subsystem ==
  In1 : Inport
  Action Port : ActionPort  ActionPortLabel=case [ 0 ]:
  To File : ToFile  Filename=CircadianProcess1.mat  MatrixName=H_L_CircardianLow_RBM_SWA  SampleTime=sampletime
  wires:
  In1/1 -> To File/1

== system PNEUMA/Respiratory System/Sleep Mechanism/Saving CircadianProcess/Switch Case Action Subsystem1 ==
  In1 : Inport
  Action Port : ActionPort  ActionPortLabel=case [ 1 ]:
  To File : ToFile  Filename=CircadianProcess2.mat  MatrixName=H_L_CircardianLow_RBM_SWA  SampleTime=sampletime
  wires:
  In1/1 -> To File/1

== system PNEUMA/Respiratory System/Sleep Mechanism/Saving CircadianProcess/Switch Case Action Subsystem2 ==
  In1 : Inport
  Action Port : ActionPort  ActionPortLabel=case [ 2 ]:
  To File : ToFile  Filename=CircadianProcess3.mat  MatrixName=H_L_CircardianLow_RBM_SWA  SampleTime=sampletime
  wires:
  In1/1 -> To File/1

== system PNEUMA/Respiratory System/Sleep Mechanism/Saving CircadianProcess/Switch Case Action Subsystem3 ==
  In1 : Inport
  Action Port : ActionPort  ActionPortLabel=default:
  To File : ToFile  Filename=CircadianProcess10.mat  MatrixName=H_L_CircardianLow_RBM_SWA  SampleTime=sampletime
  wires:
  In1/1 -> To File/1

== system PNEUMA/Respiratory System/Sleep Mechanism/Saving CircadianProcess/Switch Case Action Subsystem4 ==
  In1 : Inport
  Action Port : ActionPort  ActionPortLabel=case [ 3 ]:
  To File : ToFile  Filename=CircadianProcess4.mat  MatrixName=H_L_CircardianLow_RBM_SWA  SampleTime=sampletime
  wires:
  In1/1 -> To File/1

== system PNEUMA/Respiratory System/Sleep Mechanism/Saving CircadianProcess/Switch Case Action Subsystem5 ==
  In1 : Inport
  Action Port : ActionPort  ActionPortLabel=case [ 4 ]:
  To File : ToFile  Filename=CircadianProcess5.mat  MatrixName=H_L_CircardianLow_RBM_SWA  SampleTime=sampletime
  wires:
  In1/1 -> To File/1

== system PNEUMA/Respiratory System/Sleep Mechanism/Saving CircadianProcess/Switch Case Action Subsystem6 ==
  In1 : Inport
  Action Port : ActionPort  ActionPortLabel=case [ 5 ]:
  To File : ToFile  Filename=CircadianProcess6.mat  MatrixName=H_L_CircardianLow_RBM_SWA  SampleTime=sampletime
  wires:
  In1/1 -> To File/1

== system PNEUMA/Respiratory System/Sleep Mechanism/Saving CircadianProcess/Switch Case Action Subsystem7 ==
  In1 : Inport
  Action Port : ActionPort  ActionPortLabel=case [ 6 ]:
  To File : ToFile  Filename=CircadianProcess7.mat  MatrixName=H_L_CircardianLow_RBM_SWA  SampleTime=sampletime
  wires:
  In1/1 -> To File/1

== system PNEUMA/Respiratory System/Sleep Mechanism/Saving CircadianProcess/Switch Case Action Subsystem8 ==
  In1 : Inport
  Action Port : ActionPort  ActionPortLabel=case [ 7 ]:
  To File : ToFile  Filename=CircadianProcess8.mat  MatrixName=H_L_CircardianLow_RBM_SWA  SampleTime=sampletime
  wires:
  In1/1 -> To File/1

== system PNEUMA/Respiratory System/Sleep Mechanism/Saving CircadianProcess/Switch Case Action Subsystem9 ==
  In1 : Inport
  Action Port : ActionPort  ActionPortLabel=case [ 8 ]:
  To File : ToFile  Filename=CircadianProcess9.mat  MatrixName=H_L_CircardianLow_RBM_SWA  SampleTime=sampletime
  wires:
  In1/1 -> To File/1

== system PNEUMA/Respiratory System/Upper_Airway_Mechanism/Upper_Airway_Model/ Flow in Upper Airway ==
  C_ua Upper Airway Compliance : Inport
  P_ua Pressure in Upper Airways : Inport  Port=2
  Coefficient1 : Gain  Gain=-1  SaturateOnIntegerOverflow=on  OutDataTypeStr=Inherit: Same as input  ParamDataTypeStr=Inherit: Same as input
  Coefficient2 : Gain  SaturateOnIntegerOverflow=on  OutDataTypeStr=Inherit: Same as input  ParamDataTypeStr=Inherit: Same as input
  Constant : Constant  Value=R_trachea*10
  Integrator : Integrator  LimitOutput=on  UpperSaturationLimit=100  LowerSaturationLimit=-100
  Math Function : Math  Operator=reciprocal  SignedPower=on
  Math Function1 : Math  Operator=reciprocal  SignedPower=on
  Memory : Memory
  Product : Product  SaturateOnIntegerOverflow=on  OutDataTypeStr=Inherit: Same as first input
  Product1 : Product  SaturateOnIntegerOverflow=on  OutDataTypeStr=Inherit: Same as first input
  Sum : Sum  Inputs=|++  SaturateOnIntegerOverflow=on
  "Q_ua Upper Airway Flow " : Outport
  wires:
  Product1/1 -> Integrator/1, Memory/1
  P_ua Pressure in Upper Airways/1 -> Sum/1
  Sum/1 -> Product1/2
  C_ua Upper Airway Compliance/1 -> Math Function1/1
  Integrator/1 -> Product/1
  Product/1 -> Sum/2
  Constant/1 -> Math Function/1
  Math Function/1 -> Coefficient1/1
  Coefficient1/1 -> Product1/1
  Coefficient2/1 -> "Q_ua Upper Airway Flow "/1
  Memory/1 -> Coefficient2/1
  Math Function1/1 -> Product/2

== system PNEUMA/Respiratory System/Upper_Airway_Mechanism/Upper_Airway_Model/ Pressure in Upper Airway ==
  P_pl Pleural Pressure : Inport
  Q_la Lower Airway Flow : Inport  Port=2
  R_LA Lower Airways Resistance : Gain  Gain=R_LAW+R_L+R_CW  SaturateOnIntegerOverflow=on  OutDataTypeStr=Inherit: Same as input  ParamDataTypeStr=Inherit: Same as input
  R_LA Lower Airways Resistance1 : Gain  Gain=0.7  SaturateOnIntegerOverflow=on  OutDataTypeStr=Inherit: Same as input  ParamDataTypeStr=Inherit: Same as input
  Sum2 : Sum  SaturateOnIntegerOverflow=on
  "P_ua Upper Airway Pressure " : Outport  InitialOutput=[0]
  wires:
  Q_la Lower Airway Flow/1 -> R_LA Lower Airways Resistance/1  "Q_la Lower Airway Flow"
  P_pl Pleural Pressure/1 -> Sum2/2
  Sum2/1 -> "P_ua Upper Airway Pressure "/1
  R_LA Lower Airways Resistance/1 -> R_LA Lower Airways Resistance1/1
  R_LA Lower Airways Resistance1/1 -> Sum2/1

== system PNEUMA/Respiratory System/Upper_Airway_Mechanism/Upper_Airway_Model/Upper Airway Conductance3 ==
  C_ua_Upper_Airway_Compliance : Inport
  P_ua_Upper Airway Pressure : Inport  Port=2
  A_0_ua : Constant  Value=A_0_ua
  Fcn : Fcn  Expr="( u(5) <=u(6) )* u(1)*0  + (u(5) >0.0)* u(1) * u(2) +  ( u(5) >u(6) )* (u(5) <=0.0) * ( u(7)>=0 ) * u(7)"
  Fcn1 : Fcn  Expr=u(2) * (1+u(3)*u(4)*u(5)) *u(1)
  Gain : Gain  Gain=-1  SaturateOnIntegerOverflow=on  OutDataTypeStr=Inherit: Same as input  ParamDataTypeStr=Inherit: Same as input
  K_ua : Constant  Value=K_ua
  Math Function : Math  Operator=reciprocal  SignedPower=on
  Mux1 : Mux  Inputs=7
  Mux2 : Mux  Inputs=5
  Product : Product  SaturateOnIntegerOverflow=on  OutDataTypeStr=Inherit: Same as first input
  Saturation : Saturate  UpperLimit=10  LowerLimit=-40
  b_ua*13 : Constant  Value=13
  Y_ua_Upper Airway Conductance : Outport
  P_crit : Outport  Port=2
  wires:
  P_ua_Upper Airway Pressure/1 -> Mux1/5, Mux2/5  "P_ua"
  K_ua/1 -> Mux1/1, Mux2/1
  C_ua_Upper_Airway_Compliance/1 -> Mux1/4, Mux2/4, Product/1  "C_ua"
  b_ua*13/1 -> Mux1/3, Mux2/3, Product/2  "b_ua"
  A_0_ua/1 -> Mux1/2, Mux2/2  "A_0_ua"
  Mux1/1 -> Fcn/1
  Fcn/1 -> Y_ua_Upper Airway Conductance/1
  Fcn1/1 -> Mux1/7
  Mux2/1 -> Fcn1/1
  Gain/1 -> Saturation/1
  Product/1 -> Math Function/1
  Math Function/1 -> Gain/1
  Saturation/1 -> Mux1/6, P_crit/1

== system PNEUMA/Respiratory System/Upper_Airway_Mechanism/Upper_Airway_Model/Upper_Airway_Compliance ==
  "SI Sleep Wake State Index " : Inport
  Sleep/awake : Inport  Port=2
  % increase : Gain  Gain=35  SaturateOnIntegerOverflow=on  OutDataTypeStr=Inherit: Same as input  ParamDataTypeStr=Inherit: Same as input
  Awake Upper Airway Compliance : Constant  Value=C_ua_awake
  Fcn : Fcn  Expr="( u(1) <=0 ) * u(2) + ( u(1) >=1) * u(2) * ( 1+u(3) ) +  ( u(1) >0 ) * ( u(1) <1 ) * u(2) * ( 1+u(3)*u(1)*u(1) * ( 1- u(4)))"
  Mux1 : Mux
  S_UA : Constant  Value=0.01
  C_ua Upper Airway Compliance : Outport
  wires:
  Awake Upper Airway Compliance/1 -> Mux1/2
  "SI Sleep Wake State Index "/1 -> Mux1/1
  % increase/1 -> Mux1/3
  Mux1/1 -> Fcn/1
  Fcn/1 -> C_ua Upper Airway Compliance/1
  S_UA/1 -> % increase/1
  Sleep/awake/1 -> Mux1/4

== system PNEUMA/Cardiovascular System/Local Flow Regulation/Cerebral Circulation Regulation/Subsystem/If Action Subsystem ==
  In1 : Inport
  Action Port : ActionPort  ActionPortLabel=if(u1 == 0)
  Out1 : Outport
  wires:
  In1/1 -> Out1/1

== system PNEUMA/Cardiovascular System/Local Flow Regulation/Coronary Circulation Regulation2/Subsystem/If Action Subsystem ==
  In1 : Inport
  Action Port : ActionPort  ActionPortLabel=if(u1 == 0)
  Out1 : Outport
  wires:
  In1/1 -> Out1/1

== system PNEUMA/Cardiovascular System/Local Flow Regulation/Muscular Circulation Regulation1/Subsystem/If Action Subsystem ==
  In1 : Inport
  Action Port : ActionPort  ActionPortLabel=if(u1 == 0)
  Out1 : Outport
  wires:
  In1/1 -> Out1/1

== system PNEUMA/Cardiovascular System/SA-node and Autonomic Control/RR Interval/Saving varHeartPeriod/Switch Case Action Subsystem ==
  In1 : Inport
  Action Port : ActionPort  ActionPortLabel=case [ 0 ]:
  To File : ToFile  Filename=varHeartPeriod1.mat  MatrixName=HPsa_HPin_HPout_HP_Enable  SampleTime=0.1
  wires:
  In1/1 -> To File/1

== system PNEUMA/Cardiovascular System/SA-node and Autonomic Control/RR Interval/Saving varHeartPeriod/Switch Case Action Subsystem1 ==
  In1 : Inport
  Action Port : ActionPort  ActionPortLabel=case [ 1 ]:
  To File : ToFile  Filename=varHeartPeriod2.mat  MatrixName=HPsa_HPin_HPout_HP_Enable  SampleTime=0.1
  wires:
  In1/1 -> To File/1

== system PNEUMA/Cardiovascular System/SA-node and Autonomic Control/RR Interval/Saving varHeartPeriod/Switch Case Action Subsystem2 ==
  In1 : Inport
  Action Port : ActionPort  ActionPortLabel=case [ 2 ]:
  To File : ToFile  Filename=varHeartPeriod3.mat  MatrixName=HPsa_HPin_HPout_HP_Enable  SampleTime=0.1
  wires:
  In1/1 -> To File/1

== system PNEUMA/Cardiovascular System/SA-node and Autonomic Control/RR Interval/Saving varHeartPeriod/Switch Case Action Subsystem3 ==
  In1 : Inport
  Action Port : ActionPort  ActionPortLabel=default:
  To File : ToFile  Filename=varHeartPeriod10.mat  MatrixName=HPsa_HPin_HPout_HP_Enable  SampleTime=0.1
  wires:
  In1/1 -> To File/1

== system PNEUMA/Cardiovascular System/SA-node and Autonomic Control/RR Interval/Saving varHeartPeriod/Switch Case Action Subsystem4 ==
  In1 : Inport
  Action Port : ActionPort  ActionPortLabel=case [ 3 ]:
  To File : ToFile  Filename=varHeartPeriod4.mat  MatrixName=HPsa_HPin_HPout_HP_Enable  SampleTime=0.1
  wires:
  In1/1 -> To File/1

== system PNEUMA/Cardiovascular System/SA-node and Autonomic Control/RR Interval/Saving varHeartPeriod/Switch Case Action Subsystem5 ==
  In1 : Inport
  Action Port : ActionPort  ActionPortLabel=case [ 4 ]:
  To File : ToFile  Filename=varHeartPeriod5.mat  MatrixName=HPsa_HPin_HPout_HP_Enable  SampleTime=0.1
  wires:
  In1/1 -> To File/1

== system PNEUMA/Cardiovascular System/SA-node and Autonomic Control/RR Interval/Saving varHeartPeriod/Switch Case Action Subsystem6 ==
  In1 : Inport
  Action Port : ActionPort  ActionPortLabel=case [ 5 ]:
  To File : ToFile  Filename=varHeartPeriod6.mat  MatrixName=HPsa_HPin_HPout_HP_Enable  SampleTime=0.1
  wires:
  In1/1 -> To File/1

== system PNEUMA/Cardiovascular System/SA-node and Autonomic Control/RR Interval/Saving varHeartPeriod/Switch Case Action Subsystem7 ==
  In1 : Inport
  Action Port : ActionPort  ActionPortLabel=case [ 6 ]:
  To File : ToFile  Filename=varHeartPeriod7.mat  MatrixName=HPsa_HPin_HPout_HP_Enable  SampleTime=0.1
  wires:
  In1/1 -> To File/1

== system PNEUMA/Cardiovascular System/SA-node and Autonomic Control/RR Interval/Saving varHeartPeriod/Switch Case Action Subsystem8 ==
  In1 : Inport
  Action Port : ActionPort  ActionPortLabel=case [ 7 ]:
  To File : ToFile  Filename=varHeartPeriod8.mat  MatrixName=HPsa_HPin_HPout_HP_Enable  SampleTime=0.1
  wires:
  In1/1 -> To File/1

== system PNEUMA/Cardiovascular System/SA-node and Autonomic Control/RR Interval/Saving varHeartPeriod/Switch Case Action Subsystem9 ==
  In1 : Inport
  Action Port : ActionPort  ActionPortLabel=case [ 8 ]:
  To File : ToFile  Filename=varHeartPeriod9.mat  MatrixName=HPsa_HPin_HPout_HP_Enable  SampleTime=0.1
  wires:
  In1/1 -> To File/1

== system PNEUMA/Central Neural Control/VARIABLE RESPIRATORY RHYTHM1/Variable Breathing Period Reset/Saving BreathingPeriod/Switch Case Action Subsystem ==
  In1 : Inport
  Action Port : ActionPort  ActionPortLabel=case [ 0 ]:
  To File : ToFile  Filename=BreathingPeriod1.mat  MatrixName=BreathingPeriod  SampleTime=sampletime
  wires:
  In1/1 -> To File/1

== system PNEUMA/Central Neural Control/VARIABLE RESPIRATORY RHYTHM1/Variable Breathing Period Reset/Saving BreathingPeriod/Switch Case Action Subsystem1 ==
  In1 : Inport
  Action Port : ActionPort  ActionPortLabel=case [ 1 ]:
  To File : ToFile  Filename=BreathingPeriod2.mat  MatrixName=BreathingPeriod  SampleTime=sampletime
  wires:
  In1/1 -> To File/1

== system PNEUMA/Central Neural Control/VARIABLE RESPIRATORY RHYTHM1/Variable Breathing Period Reset/Saving BreathingPeriod/Switch Case Action Subsystem2 ==
  In1 : Inport
  Action Port : ActionPort  ActionPortLabel=case [ 2 ]:
  To File : ToFile  Filename=BreathingPeriod3.mat  MatrixName=BreathingPeriod  SampleTime=sampletime
  wires:
  In1/1 -> To File/1

== system PNEUMA/Central Neural Control/VARIABLE RESPIRATORY RHYTHM1/Variable Breathing Period Reset/Saving BreathingPeriod/Switch Case Action Subsystem3 ==
  In1 : Inport
  Action Port : ActionPort  ActionPortLabel=default:
  To File : ToFile  Filename=BreathingPeriod10.mat  MatrixName=BreathingPeriod  SampleTime=sampletime
  wires:
  In1/1 -> To File/1

== system PNEUMA/Central Neural Control/VARIABLE RESPIRATORY RHYTHM1/Variable Breathing Period Reset/Saving BreathingPeriod/Switch Case Action Subsystem4 ==
  In1 : Inport
  Action Port : ActionPort  ActionPortLabel=case [ 3 ]:
  To File : ToFile  Filename=BreathingPeriod4.mat  MatrixName=BreathingPeriod  SampleTime=sampletime
  wires:
  In1/1 -> To File/1

== system PNEUMA/Central Neural Control/VARIABLE RESPIRATORY RHYTHM1/Variable Breathing Period Reset/Saving BreathingPeriod/Switch Case Action Subsystem5 ==
  In1 : Inport
  Action Port : ActionPort  ActionPortLabel=case [ 4 ]:
  To File : ToFile  Filename=BreathingPeriod5.mat  MatrixName=BreathingPeriod  SampleTime=sampletime
  wires:
  In1/1 -> To File/1

== system PNEUMA/Central Neural Control/VARIABLE RESPIRATORY RHYTHM1/Variable Breathing Period Reset/Saving BreathingPeriod/Switch Case Action Subsystem6 ==
  In1 : Inport
  Action Port : ActionPort  ActionPortLabel=case [ 5 ]:
  To File : ToFile  Filename=BreathingPeriod6.mat  MatrixName=BreathingPeriod  SampleTime=sampletime
  wires:
  In1/1 -> To File/1

== system PNEUMA/Central Neural Control/VARIABLE RESPIRATORY RHYTHM1/Variable Breathing Period Reset/Saving BreathingPeriod/Switch Case Action Subsystem7 ==
  In1 : Inport
  Action Port : ActionPort  ActionPortLabel=case [ 6 ]:
  To File : ToFile  Filename=BreathingPeriod7.mat  MatrixName=BreathingPeriod  SampleTime=sampletime
  wires:
  In1/1 -> To File/1

== system PNEUMA/Central Neural Control/VARIABLE RESPIRATORY RHYTHM1/Variable Breathing Period Reset/Saving BreathingPeriod/Switch Case Action Subsystem8 ==
  In1 : Inport
  Action Port : ActionPort  ActionPortLabel=case [ 7 ]:
  To File : ToFile  Filename=BreathingPeriod8.mat  MatrixName=BreathingPeriod  SampleTime=sampletime
  wires:
  In1/1 -> To File/1

== system PNEUMA/Central Neural Control/VARIABLE RESPIRATORY RHYTHM1/Variable Breathing Period Reset/Saving BreathingPeriod/Switch Case Action Subsystem9 ==
  In1 : Inport
  Action Port : ActionPort  ActionPortLabel=case [ 8 ]:
  To File : ToFile  Filename=BreathingPeriod9.mat  MatrixName=BreathingPeriod  SampleTime=sampletime
  wires:
  In1/1 -> To File/1

== system PNEUMA/Central Neural Control/VENTILATORY DRIVE (chemical)/Dynamic Drive/Saving stpres/Switch Case Action Subsystem ==
  In1 : Inport
  Action Port : ActionPort  ActionPortLabel=case [ 0 ]:
  To File : ToFile  Filename=stpres1.mat  MatrixName=tuzy  SampleTime=sampletime
  wires:
  In1/1 -> To File/1

== system PNEUMA/Central Neural Control/VENTILATORY DRIVE (chemical)/Dynamic Drive/Saving stpres/Switch Case Action Subsystem1 ==
  In1 : Inport
  Action Port : ActionPort  ActionPortLabel=case [ 1 ]:
  To File : ToFile  Filename=stpres2.mat  MatrixName=tuzy  SampleTime=sampletime
  wires:
  In1/1 -> To File/1

== system PNEUMA/Central Neural Control/VENTILATORY DRIVE (chemical)/Dynamic Drive/Saving stpres/Switch Case Action Subsystem2 ==
  In1 : Inport
  Action Port : ActionPort  ActionPortLabel=case [ 2 ]:
  To File : ToFile  Filename=stpres3.mat  MatrixName=tuzy  SampleTime=sampletime
  wires:
  In1/1 -> To File/1

== system PNEUMA/Central Neural Control/VENTILATORY DRIVE (chemical)/Dynamic Drive/Saving stpres/Switch Case Action Subsystem3 ==
  In1 : Inport
  Action Port : ActionPort  ActionPortLabel=default:
  To File : ToFile  Filename=stpres10.mat  MatrixName=tuzy  SampleTime=sampletime
  wires:
  In1/1 -> To File/1

== system PNEUMA/Central Neural Control/VENTILATORY DRIVE (chemical)/Dynamic Drive/Saving stpres/Switch Case Action Subsystem4 ==
  In1 : Inport
  Action Port : ActionPort  ActionPortLabel=case [ 3 ]:
  To File : ToFile  Filename=stpres4.mat  MatrixName=tuzy  SampleTime=sampletime
  wires:
  In1/1 -> To File/1

== system PNEUMA/Central Neural Control/VENTILATORY DRIVE (chemical)/Dynamic Drive/Saving stpres/Switch Case Action Subsystem5 ==
  In1 : Inport
  Action Port : ActionPort  ActionPortLabel=case [ 4 ]:
  To File : ToFile  Filename=stpres5.mat  MatrixName=tuzy  SampleTime=sampletime
  wires:
  In1/1 -> To File/1

== system PNEUMA/Central Neural Control/VENTILATORY DRIVE (chemical)/Dynamic Drive/Saving stpres/Switch Case Action Subsystem6 ==
  In1 : Inport
  Action Port : ActionPort  ActionPortLabel=case [ 5 ]:
  To File : ToFile  Filename=stpres6.mat  MatrixName=tuzy  SampleTime=sampletime
  wires:
  In1/1 -> To File/1

== system PNEUMA/Central Neural Control/VENTILATORY DRIVE (chemical)/Dynamic Drive/Saving stpres/Switch Case Action Subsystem7 ==
  In1 : Inport
  Action Port : ActionPort  ActionPortLabel=case [ 6 ]:
  To File : ToFile  Filename=stpres7.mat  MatrixName=tuzy  SampleTime=sampletime
  wires:
  In1/1 -> To File/1

== system PNEUMA/Central Neural Control/VENTILATORY DRIVE (chemical)/Dynamic Drive/Saving stpres/Switch Case Action Subsystem8 ==
  In1 : Inport
  Action Port : ActionPort  ActionPortLabel=case [ 7 ]:
  To File : ToFile  Filename=stpres8.mat  MatrixName=tuzy  SampleTime=sampletime
  wires:
  In1/1 -> To File/1

== system PNEUMA/Central Neural Control/VENTILATORY DRIVE (chemical)/Dynamic Drive/Saving stpres/Switch Case Action Subsystem9 ==
  In1 : Inport
  Action Port : ActionPort  ActionPortLabel=case [ 8 ]:
  To File : ToFile  Filename=stpres9.mat  MatrixName=tuzy  SampleTime=sampletime
  wires:
  In1/1 -> To File/1

== system PNEUMA/Respiratory System/Gas Exchange/DEAD SPACE/CO2 DEAD SPACE/Pd(1)CO2 ==
  PICO2 : Inport
  Flow : Inport  Port=2
  Pd(2)CO2 : Inport  Port=3
  1/Vdead1 : Gain  Gain=1/Vdead1  SaturateOnIntegerOverflow=on  OutDataTypeStr=Inherit: Same as input  ParamDataTypeStr=Inherit: Same as input
  Abs (v.t) : Abs
  Integrator : Integrator  InitialCondition=Dead1CO2IC
  Product : Product  InputSameDT=on  SaturateOnIntegerOverflow=on  OutDataTypeStr=Inherit: Same as first input
  Sum : Sum  Inputs=-+  InputSameDT=on  SaturateOnIntegerOverflow=on  OutDataTypeStr=Inherit: Same as first input
  Switch : Switch
  Pd(1)CO2 : Outport
  tag scope: Dead1CO2IC=global
  wires:
  Flow/1 -> Abs (v.t)/1, Switch/2
  Abs (v.t)/1 -> Product/2
  Switch/1 -> Sum/2
  Product/1 -> 1/Vdead1/1
  1/Vdead1/1 -> Integrator/1
  Integrator/1 -> [Dead1CO2IC], Pd(1)CO2/1, Sum/1
  Sum/1 -> Product/1
  PICO2/1 -> Switch/1
  Pd(2)CO2/1 -> Switch/3
